simulink model "MyComplexModel_V13R2023a"  (R2023a)
settings: Solver=ode23tb  StartTime=0.0  StopTime=30  FixedStep=0.001  MaxStep=0.001  RelTol=1e-6
values from neighbouring files (symbols this model uses):
  alpha_IS = 30 / (V30_IS.^beta_IS)    [run_one_case_conditional_sampling_pediatric_noVAD_linear.m]    (also in run_one_case_pediatric_noVAD_linear.m)
  alpha_LA = 30 / (V30_LA.^beta_LA)    [run_one_case_conditional_sampling_pediatric_noVAD_linear.m]    (also in run_one_case_pediatric_noVAD_linear.m)
  alpha_LV = 30 / (V30_LV.^beta_LV)    [run_one_case_conditional_sampling_pediatric_noVAD_linear.m]    (also in run_one_case_pediatric_noVAD_linear.m)
  alpha_RA = 30 / (V30_RA.^beta_RA)    [run_one_case_conditional_sampling_pediatric_noVAD_linear.m]    (also in run_one_case_pediatric_noVAD_linear.m)
  alpha_RV = 30 / (V30_RV.^beta_RV)    [run_one_case_conditional_sampling_pediatric_noVAD_linear.m]    (also in run_one_case_pediatric_noVAD_linear.m)
  beta_IS = (log(Pm_IS / 30)) / (log(Vm_IS / V30_IS))    [run_one_case_conditional_sampling_pediatric_noVAD_linear.m]    (also in run_one_case_pediatric_noVAD_linear.m)
  beta_LA = (log(Pm_LA / 30)) / (log(Vm_LA / V30_LA))    [run_one_case_conditional_sampling_pediatric_noVAD_linear.m]    (also in run_one_case_pediatric_noVAD_linear.m)
  beta_LV = (log(Pm_LV / 30)) / (log(Vm_LV / V30_LV))    [run_one_case_conditional_sampling_pediatric_noVAD_linear.m]    (also in run_one_case_pediatric_noVAD_linear.m)
  beta_RA = (log(Pm_RA / 30)) / (log(Vm_RA / V30_RA))    [run_one_case_conditional_sampling_pediatric_noVAD_linear.m]    (also in run_one_case_pediatric_noVAD_linear.m)
  beta_RV = (log(Pm_RV / 30)) / (log(Vm_RV / V30_RV))    [run_one_case_conditional_sampling_pediatric_noVAD_linear.m]    (also in run_one_case_pediatric_noVAD_linear.m)
  C_can_H = 5e-6    (= 5e-06)    [run_one_case_conditional_sampling_pediatric_noVAD_linear.m]    (also in run_one_case_pediatric_noVAD_linear.m)
  Cla = 1.6 * 2    (= 3.2)    [run_one_case_conditional_sampling_pediatric_noVAD_linear.m]    (also in run_one_case_pediatric_noVAD_linear.m)
  Cpulmart = SV_RV / (sPAP - dPAP) * 0.65    [run_one_case_conditional_sampling_pediatric_noVAD_linear.m]    (also in run_one_case_pediatric_noVAD_linear.m = 0.830555555556)
  Cpulmven = Cpulm - Cpulmart    [run_one_case_conditional_sampling_pediatric_noVAD_linear.m]    (also in run_one_case_pediatric_noVAD_linear.m)
  Cra = 4.2 * 2    (= 8.4)    [run_one_case_conditional_sampling_pediatric_noVAD_linear.m]    (also in run_one_case_pediatric_noVAD_linear.m)
  Csysart = SV_LV / (SAP - DAP)    [run_one_case_conditional_sampling_pediatric_noVAD_linear.m]    (also in run_one_case_pediatric_noVAD_linear.m = 0.589743589744)
  Csysven = Csys - Csysart    [run_one_case_conditional_sampling_pediatric_noVAD_linear.m]    (also in run_one_case_pediatric_noVAD_linear.m)
  DE = 2 * 0    (= 0)    [run_one_case_conditional_sampling_pediatric_noVAD_linear.m]    (also in run_one_case_pediatric_noVAD_linear.m)
  DR = 3 * 0    (= 0)    [run_one_case_conditional_sampling_pediatric_noVAD_linear.m]    (also in run_one_case_pediatric_noVAD_linear.m)
  DTs = 3 * 0    (= 0)    [run_one_case_conditional_sampling_pediatric_noVAD_linear.m]    (also in run_one_case_pediatric_noVAD_linear.m)
  DTv = 0.5 * 0    (= 0)    [run_one_case_conditional_sampling_pediatric_noVAD_linear.m]    (also in run_one_case_pediatric_noVAD_linear.m)
  DV = 5 * 0    (= 0)    [run_one_case_conditional_sampling_pediatric_noVAD_linear.m]    (also in run_one_case_pediatric_noVAD_linear.m)
  Emax_LV = 0.5    [run_one_case_conditional_sampling_pediatric_noVAD_linear.m]    (also in run_one_case_pediatric_noVAD_linear.m)
  Emax_RV = 0.5    [run_one_case_conditional_sampling_pediatric_noVAD_linear.m]    (also in run_one_case_pediatric_noVAD_linear.m)
  Emin_LV = -0.5    [run_one_case_conditional_sampling_pediatric_noVAD_linear.m]    (also in run_one_case_pediatric_noVAD_linear.m)
  Emin_RV = -0.5    [run_one_case_conditional_sampling_pediatric_noVAD_linear.m]    (also in run_one_case_pediatric_noVAD_linear.m)
  ESP_LA = LAP * 1.2    [run_one_case_conditional_sampling_pediatric_noVAD_linear.m]    (also in run_one_case_pediatric_noVAD_linear.m = 22.8)
  ESP_LV = k_ESP_LV * SAP    [run_one_case_conditional_sampling_pediatric_noVAD_linear.m]    (also in run_one_case_pediatric_noVAD_linear.m)
  ESP_RA = CVP * 1.2    [run_one_case_conditional_sampling_pediatric_noVAD_linear.m]    (also in run_one_case_pediatric_noVAD_linear.m = 12)
  ESP_RV = k_ESP_RV * sPAP    [run_one_case_conditional_sampling_pediatric_noVAD_linear.m]    (also in run_one_case_pediatric_noVAD_linear.m)
  ESV_LA = EDV_LA - SV_LA    [run_one_case_conditional_sampling_pediatric_noVAD_linear.m]    (also in run_one_case_pediatric_noVAD_linear.m = 59.75)
  ESV_LV = get_required_scalar(sample_row, {'ESVLV', 'ESV_LV'})    [run_one_case_conditional_sampling_pediatric_noVAD_linear.m]    (also in run_one_case_pediatric_noVAD_linear.m = 76)
  ESV_RA = EDV_RA - SV_RA    [run_one_case_conditional_sampling_pediatric_noVAD_linear.m]    (also in run_one_case_pediatric_noVAD_linear.m = 30.05)
  ESV_RV = get_required_scalar(sample_row, {'ESVRV', 'ESV_RV'})    [run_one_case_conditional_sampling_pediatric_noVAD_linear.m]    (also in run_one_case_pediatric_noVAD_linear.m = 40)
  GaE = 0.012    [run_one_case_conditional_sampling_pediatric_noVAD_linear.m]    (also in run_one_case_pediatric_noVAD_linear.m)
  GaR = 0.1    [run_one_case_conditional_sampling_pediatric_noVAD_linear.m]    (also in run_one_case_pediatric_noVAD_linear.m)
  GaTs = 0.015    [run_one_case_conditional_sampling_pediatric_noVAD_linear.m]    (also in run_one_case_pediatric_noVAD_linear.m)
  GaTv = 0.028    [run_one_case_conditional_sampling_pediatric_noVAD_linear.m]    (also in run_one_case_pediatric_noVAD_linear.m)
  GaV = 9.29    [run_one_case_conditional_sampling_pediatric_noVAD_linear.m]    (also in run_one_case_pediatric_noVAD_linear.m)
  GpE = 0    [run_one_case_conditional_sampling_pediatric_noVAD_linear.m]    (also in run_one_case_pediatric_noVAD_linear.m)
  GpR = 0.33    [run_one_case_conditional_sampling_pediatric_noVAD_linear.m]    (also in run_one_case_pediatric_noVAD_linear.m)
  GpTs = 0    [run_one_case_conditional_sampling_pediatric_noVAD_linear.m]    (also in run_one_case_pediatric_noVAD_linear.m)
  GpTv = 0.25    [run_one_case_conditional_sampling_pediatric_noVAD_linear.m]    (also in run_one_case_pediatric_noVAD_linear.m)
  GpV = 0    [run_one_case_conditional_sampling_pediatric_noVAD_linear.m]    (also in run_one_case_pediatric_noVAD_linear.m)
  hr = get_required_scalar(sample_row, {'hr'})    [run_one_case_conditional_sampling_pediatric_noVAD_linear.m]    (also in run_one_case_pediatric_noVAD_linear.m = 112)
  kELV = (Emax_LV - Emin_LV) / (4 * SE0)    (= 0.25)    [run_one_case_conditional_sampling_pediatric_noVAD_linear.m]    (also in run_one_case_pediatric_noVAD_linear.m)
  kERV = (Emax_RV - Emin_RV) / (4 * SE0)    (= 0.25)    [run_one_case_conditional_sampling_pediatric_noVAD_linear.m]    (also in run_one_case_pediatric_noVAD_linear.m)
  kR = (Rmax - Rmin) / (4 * SR0)    (= 0.174809457508)    [run_one_case_conditional_sampling_pediatric_noVAD_linear.m]    (also in run_one_case_pediatric_noVAD_linear.m)
  kT = (Tmax - Tmin) / (4 * ST0)    (= 0.252)    [run_one_case_conditional_sampling_pediatric_noVAD_linear.m]    (also in run_one_case_pediatric_noVAD_linear.m)
  kV = (Vmax - Vmin) / (4 * SV0) / 100    (= 1.75)    [run_one_case_conditional_sampling_pediatric_noVAD_linear.m]    (also in run_one_case_pediatric_noVAD_linear.m)
  L = 1e-6    (= 1e-06)    [Simulink_vars_code.m]    (also in run_one_case_conditional_sampling_pediatric_noVAD_linear.m; run_one_case_pediatric_noVAD_linear.m)
  Lav = Lav / fct    (= 5.64234254909e-06)    [run_one_case_conditional_sampling_pediatric_noVAD_linear.m]    (also in run_one_case_pediatric_noVAD_linear.m)
  Lmv = Lmv / fct    (= 3.13989149577e-06)    [run_one_case_conditional_sampling_pediatric_noVAD_linear.m]    (also in run_one_case_pediatric_noVAD_linear.m)
  Lpv = Lpv / fct    (= 5.14307516405e-06)    [run_one_case_conditional_sampling_pediatric_noVAD_linear.m]    (also in run_one_case_pediatric_noVAD_linear.m)
  Ltv = Ltv / fct    (= 2.29209519806e-06)    [run_one_case_conditional_sampling_pediatric_noVAD_linear.m]    (also in run_one_case_pediatric_noVAD_linear.m)
  mcfp = CO / 60 * Rsysven + CVP    [run_one_case_conditional_sampling_pediatric_noVAD_linear.m]    (also in run_one_case_pediatric_noVAD_linear.m)
  Poffset_IS = Poffset_LV    (= 0)    [run_one_case_conditional_sampling_pediatric_noVAD_linear.m]    (also in run_one_case_pediatric_noVAD_linear.m)
  Poffset_LA = 0    [run_one_case_conditional_sampling_pediatric_noVAD_linear.m]    (also in run_one_case_pediatric_noVAD_linear.m)
  Poffset_LV = 0    [run_one_case_conditional_sampling_pediatric_noVAD_linear.m]    (also in run_one_case_pediatric_noVAD_linear.m)
  Poffset_RA = 0    [run_one_case_conditional_sampling_pediatric_noVAD_linear.m]    (also in run_one_case_pediatric_noVAD_linear.m)
  Poffset_RV = 0    [run_one_case_conditional_sampling_pediatric_noVAD_linear.m]    (also in run_one_case_pediatric_noVAD_linear.m)
  Ps_IS = Ps_LV    [run_one_case_conditional_sampling_pediatric_noVAD_linear.m]    (also in run_one_case_pediatric_noVAD_linear.m)
  Ps_LA = ESP_LA    [run_one_case_conditional_sampling_pediatric_noVAD_linear.m]    (also in run_one_case_pediatric_noVAD_linear.m = 22.8)
  Ps_LV = ESP_LV    [run_one_case_conditional_sampling_pediatric_noVAD_linear.m]    (also in run_one_case_pediatric_noVAD_linear.m)
  Ps_RA = ESP_RA    [run_one_case_conditional_sampling_pediatric_noVAD_linear.m]    (also in run_one_case_pediatric_noVAD_linear.m = 12)
  Ps_RV = ESP_RV    [run_one_case_conditional_sampling_pediatric_noVAD_linear.m]    (also in run_one_case_pediatric_noVAD_linear.m)
  R = 1e-6    (= 1e-06)    [Simulink_vars_code.m]    (also in run_one_case_conditional_sampling_pediatric_noVAD_linear.m; run_one_case_pediatric_noVAD_linear.m)
  Rdir_AV = 0.00375    [run_one_case_conditional_sampling_pediatric_noVAD_linear.m]    (also in run_one_case_pediatric_noVAD_linear.m)
  Rdir_MV = 0.0075    [run_one_case_conditional_sampling_pediatric_noVAD_linear.m]    (also in run_one_case_pediatric_noVAD_linear.m)
  Rdir_PV = 0.00375    [run_one_case_conditional_sampling_pediatric_noVAD_linear.m]    (also in run_one_case_pediatric_noVAD_linear.m)
  Rdir_TV = 0.00375    [run_one_case_conditional_sampling_pediatric_noVAD_linear.m]    (also in run_one_case_pediatric_noVAD_linear.m)
  Rinv_AV = 50    [run_one_case_conditional_sampling_pediatric_noVAD_linear.m]    (also in run_one_case_pediatric_noVAD_linear.m)
  Rinv_MV = 50    [run_one_case_conditional_sampling_pediatric_noVAD_linear.m]    (also in run_one_case_pediatric_noVAD_linear.m)
  Rinv_PV = 50    [run_one_case_conditional_sampling_pediatric_noVAD_linear.m]    (also in run_one_case_pediatric_noVAD_linear.m)
  Rinv_TV = 50    [run_one_case_conditional_sampling_pediatric_noVAD_linear.m]    (also in run_one_case_pediatric_noVAD_linear.m)
  Rmax = (Rsp_max * Rep_max) / (Rsp_max + Rep_max)    (= 1.3359375)    [run_one_case_conditional_sampling_pediatric_noVAD_linear.m]    (also in run_one_case_pediatric_noVAD_linear.m)
  Rmin = (Rsp_min * Rep_min) / (Rsp_min + Rep_min)    (= 0.636699669967)    [run_one_case_conditional_sampling_pediatric_noVAD_linear.m]    (also in run_one_case_pediatric_noVAD_linear.m)
  rpm = 5500    [run_one_case_conditional_sampling_pediatric_noVAD_linear.m]    (also in run_one_case_pediatric_noVAD_linear.m)
  Rpulmart = k_Rpulmart * Rtotpulm    [run_one_case_conditional_sampling_pediatric_noVAD_linear.m]    (also in run_one_case_pediatric_noVAD_linear.m)
  Rpulmven = Rtotpulm - Rpulmart    [run_one_case_conditional_sampling_pediatric_noVAD_linear.m]    (also in run_one_case_pediatric_noVAD_linear.m)
  Rsysart = Rtotsys - Rsysven    [run_one_case_conditional_sampling_pediatric_noVAD_linear.m]    (also in run_one_case_pediatric_noVAD_linear.m)
  Rsysven = k_Rsysven * CO0 / CO    [run_one_case_conditional_sampling_pediatric_noVAD_linear.m]    (also in run_one_case_pediatric_noVAD_linear.m)
  st_a = 0    [conditional_sampling_generate_patients.m]    (also in run_one_case_conditional_sampling_pediatric_noVAD_linear.m; run_one_case_pediatric_noVAD_linear.m)
  st_v = 0    [conditional_sampling_generate_patients.m]    (also in run_one_case_conditional_sampling_pediatric_noVAD_linear.m; run_one_case_pediatric_noVAD_linear.m)
  st_VAD = 0    [conditional_sampling_generate_patients.m]    (also in run_one_case_conditional_sampling_pediatric_noVAD_linear.m; run_one_case_pediatric_noVAD_linear.m)
  st_VADtype = 0    [run_one_case_conditional_sampling_pediatric_noVAD_linear.m]    (also in run_one_case_pediatric_noVAD_linear.m)
  TauE = 1.5    [run_one_case_conditional_sampling_pediatric_noVAD_linear.m]    (also in run_one_case_pediatric_noVAD_linear.m)
  TauR = 1.5    [run_one_case_conditional_sampling_pediatric_noVAD_linear.m]    (also in run_one_case_pediatric_noVAD_linear.m)
  TauTs = 1.8    [run_one_case_conditional_sampling_pediatric_noVAD_linear.m]    (also in run_one_case_pediatric_noVAD_linear.m)
  TauTv = 0.8    [run_one_case_conditional_sampling_pediatric_noVAD_linear.m]    (also in run_one_case_pediatric_noVAD_linear.m)
  TauV = 10    [run_one_case_conditional_sampling_pediatric_noVAD_linear.m]    (also in run_one_case_pediatric_noVAD_linear.m)
  Te = Tresp - Ti    (= 3)    [run_one_case_conditional_sampling_pediatric_noVAD_linear.m]    (also in run_one_case_pediatric_noVAD_linear.m)
  Ti = 2    [run_one_case_conditional_sampling_pediatric_noVAD_linear.m]    (also in run_one_case_pediatric_noVAD_linear.m)
  Tmax = 1.308    [run_one_case_conditional_sampling_pediatric_noVAD_linear.m]    (also in run_one_case_pediatric_noVAD_linear.m)
  Tmin = 0.3    [run_one_case_conditional_sampling_pediatric_noVAD_linear.m]    (also in run_one_case_pediatric_noVAD_linear.m)
  Tresp = 5    [run_one_case_conditional_sampling_pediatric_noVAD_linear.m]    (also in run_one_case_pediatric_noVAD_linear.m)
  V0_LA = 0    [run_one_case_conditional_sampling_pediatric_noVAD_linear.m]    (also in run_one_case_pediatric_noVAD_linear.m)
  V0_LV = 0    [run_one_case_conditional_sampling_pediatric_noVAD_linear.m]    (also in run_one_case_pediatric_noVAD_linear.m)
  V0_RA = 0    [run_one_case_conditional_sampling_pediatric_noVAD_linear.m]    (also in run_one_case_pediatric_noVAD_linear.m)
  V0_RV = 0    [run_one_case_conditional_sampling_pediatric_noVAD_linear.m]    (also in run_one_case_pediatric_noVAD_linear.m)
  Vd_IS = Vd_LV * 0.1    (= 0)    [run_one_case_conditional_sampling_pediatric_noVAD_linear.m]    (also in run_one_case_pediatric_noVAD_linear.m)
  Vd_LA = 0    [run_one_case_conditional_sampling_pediatric_noVAD_linear.m]    (also in run_one_case_pediatric_noVAD_linear.m)
  Vd_LV = 0    [run_one_case_conditional_sampling_pediatric_noVAD_linear.m]    (also in run_one_case_pediatric_noVAD_linear.m)
  Vd_RA = 0    [run_one_case_conditional_sampling_pediatric_noVAD_linear.m]    (also in run_one_case_pediatric_noVAD_linear.m)
  Vd_RV = 0    [run_one_case_conditional_sampling_pediatric_noVAD_linear.m]    (also in run_one_case_pediatric_noVAD_linear.m)
  Vmax = Vusv_max + Vuev_max    (= 2846)    [run_one_case_conditional_sampling_pediatric_noVAD_linear.m]    (also in run_one_case_pediatric_noVAD_linear.m)
  Vmin = Vusv_min + Vuev_min    (= 2146)    [run_one_case_conditional_sampling_pediatric_noVAD_linear.m]    (also in run_one_case_pediatric_noVAD_linear.m)
  Vs_IS = Vs_LV * 0.1    [run_one_case_conditional_sampling_pediatric_noVAD_linear.m]    (also in run_one_case_pediatric_noVAD_linear.m = 11.4)
  Vs_LA = EDV_LA + 5    [run_one_case_conditional_sampling_pediatric_noVAD_linear.m]    (also in run_one_case_pediatric_noVAD_linear.m = 69.35)
  Vs_LV = EDV_LV + 15    [run_one_case_conditional_sampling_pediatric_noVAD_linear.m]    (also in run_one_case_pediatric_noVAD_linear.m = 114)
  Vs_RA = EDV_RA + 5    [run_one_case_conditional_sampling_pediatric_noVAD_linear.m]    (also in run_one_case_pediatric_noVAD_linear.m = 39.65)
  Vs_RV = EDV_RV + 15    [run_one_case_conditional_sampling_pediatric_noVAD_linear.m]    (also in run_one_case_pediatric_noVAD_linear.m = 78)
  Vusv_pulm_ven = k_Vusv_pulm_ven * Vusv_pulm    [run_one_case_conditional_sampling_pediatric_noVAD_linear.m]    (also in run_one_case_pediatric_noVAD_linear.m)
  Vusv_sys_ven = k_Vusv_sys_ven * Vusv_sys    [run_one_case_conditional_sampling_pediatric_noVAD_linear.m]    (also in run_one_case_pediatric_noVAD_linear.m)
undefined symbols (not defined in the file or in its folder): magnitude
libraries: spsMeanLib x9, spsMeanVariableFrequencyLib x5, simulink x3, dspsigops x1
(part 1 of 2)
settings Model: Creator=luger  LastModifiedBy=Admin
settings DataIOCC: ExternalInput=getinputstruct(op1)  InitialState=getstatestruct(op1)  SaveFormat=Array  DatasetSignalFormat=timetable
settings RTWCC: GPUComputeCapability=5.0

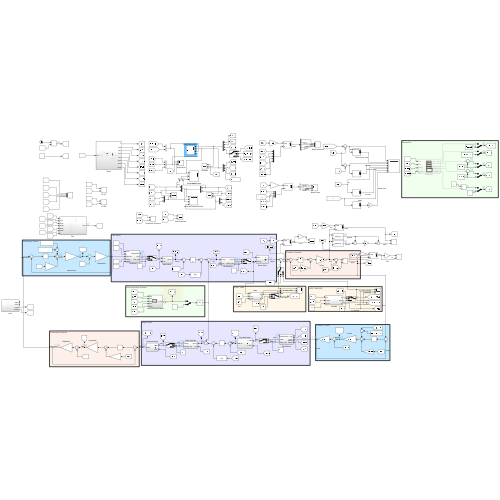
[thumbnail: Simulink's stored preview of the top-level diagram]
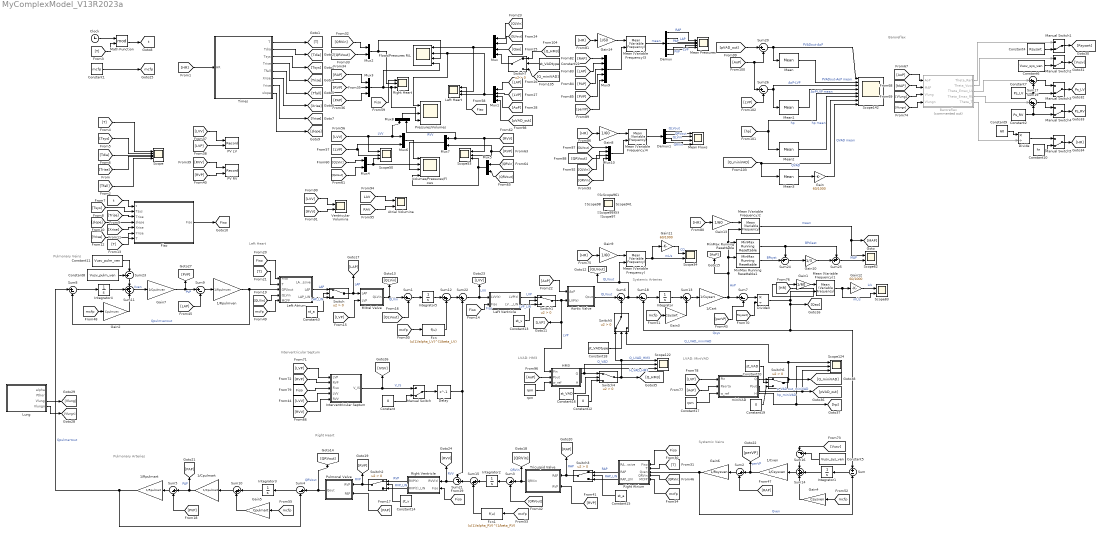
== system MyComplexModel_V13R2023a ==
  note: LVAD: MiniVAD
  note: LVAD: HM3
  note: Interventricular Septum
  note: Baroreflex
  note: Pulmonary Veins
  note: Pulmonary Arteries
  note: Systemic Veins
  note: Systemic Arteries
  note: Right Heart
  note: Left Heart
  1/Cart : Gain  Gain=1/Csysart
  1/Cpulmart : Gain  Gain=1/Cpulmart
  1/Cven : Gain  Gain=1/Csysven
  1/Rpulmart : Gain  Gain=1/Rpulmart
  1/Rpulmven : Gain  Gain=1/Rpulmven
  Aortic Valve : Subsystem
  Atrial Volumina : Scope  NumInputPorts=2
  Baroreflex : Subsystem  Commented=on
  Clock : Clock
  Constant : Constant  Value=0
  Constant1 : Constant  Value=mcfp
  Constant10 : Constant  Value=hr
  Constant11 : Constant  Value=Vusv_pulm_ven
  Constant12 : Constant  Value=0
  Constant13 : Constant  Value=st_v
  Constant14 : Constant  Value=st_v
  Constant15 : Constant  Value=st_a
  Constant16 : Constant  Value=st_VAD
  Constant17 : Constant  Value=rpm
  Constant18 : Constant  Value=st_VADtype
  Constant19 : Constant  Value=0
  Constant2 : Constant  Value=Ps_RV
  Constant20 : Constant  Value=st_VAD
  Constant21 : Constant  Value=st_VADtype
  Constant3 : Constant  Value=st_a
  Constant4 : Constant  Value=Rsysart
  Constant5 : Constant  Value=Vusv_sys_ven
  Constant6 : Constant  Value=Vusv_sys_ven
  Constant7 : Constant  Value=Ps_LV
  Constant8 : Constant  Value=Vusv_pulm_ven
  Constant9 : Constant  Value=60
  Delay : Delay  DelayLength=1  InitialCondition=0
  Demux : Demux  Outputs=5
  Demux1 : Demux
  Divide : Product  Inputs=*/
  Divide3 : Product  Inputs=*/
  Fcn : Fcn  Expr=(u(1)/alpha_LV)^(1/beta_LV)
  Fcn1 : Fcn  Expr=(u(1)/alpha_RV)^(1/beta_RV)
  Fiso : Subsystem
  Flows/Pressures R/L : Scope  NumInputPorts=4
  Gain : Gain  Gain=60/1000
  Gain{1,8..9,13..14} (5 alike) : Gain  Gain=1/60
  Gain10 : Gain  Gain=1/3
  Gain11 : Gain  Gain=60/1000
  Gain12 : Gain  Gain=60/1000
  Gain2 : Gain  Gain=Cpulmven
  Gain3 : Gain  Gain=Csysart
  Gain4 : Gain  Gain=Csysven
  Gain5 : Gain  Gain=Cpulmart
  Gain6 : Gain  Gain=1/Rsysven
  Gain7 : Gain  Gain=1/Cpulmven
  HM3 : Subsystem
  Integrator{,1..5} (6 alike) : Integrator
  Interventricular Septum : Subsystem
  Left Atrium : Subsystem
  Left Heart : Scope  NumInputPorts=3
  Left Ventricle : Subsystem
  Lung : Subsystem
  Manual Switch{,1..5} (6 alike) : ManualSwitch  CurrentSetting=0
  Math Function : Math  Operator=mod
  Mean{,1..3} (4 alike) : spsMeanLib/Mean  Freq=hr/60  Vinit=0  Ts=0
  Mean (Variable Frequency){,1..4} (5 alike) : spsMeanVariableFrequencyLib/Mean (Variable Frequency)  Finit=hr/60  Fmin=40/60  Vinit=0  Ts=0
      settings: LibrarySourceBlock=|
      | sps_lib/Sensors and Measurements/Mean
      | (Variable Frequency)
  Mean Flows : Scope  NumInputPorts=4
  Mean Pressures : Scope  NumInputPorts=5
  MinMax Running Resettable : simulink/Math Operations/MinMax Running Resettable  Function=min  vinit=80
  MinMax Running Resettable1 : simulink/Math Operations/MinMax Running Resettable  Function=max  vinit=2
  Mitral Valve : Subsystem
  Mux : Mux
  Mux1 : Mux
  Mux10 : Mux
  Mux{2,4..8} (6 alike) : Mux  Inputs=2
  Mux3 : Mux  Inputs=3
  Mux9 : Mux  Inputs=5
  PV LV : Record  FileSettingsInternal="{\"entries\":[{\"content\":{\"excelSettings\":{\"content\":{},\"type\":\"Streamout.ExcelSettings\"}},\"type\":\"Streamout.FileSettingStorage\",\"uuid\":\"\"}],\"packageUris\":[\"http:\\/\\/schema.mathworks.com\\/mf0\\/streamout_blocks\\/R2020a\"],\"version\":\"1.0\"}"  Layout=[1 1]  SignalsInternal="{\"entries\":[{\"content\":{\"signals\":[{\"content\":{\"blockPath\":[],\"dimensions\":[1],\"domain\":\"\",\"lineColor\":\"#64d413\",\"port\":1,\"sid\":[\"\"],\"signalID\":12905,\"signalName\":\"From37\"},\"type\":\"RecordBlkView.Signal\",\"uuid\":\"\"},{\"content\":{\"blockPath\":[],\"dimensions\":[1],\"domain\":\"\",\"lineColor\":\"#ff13a6\",\"port\":2,\"sid\":[\"\"],\"signalID\":12909,\"signalName\":\"From38\"},\"type\":\"RecordBlkView.Signal\",\"uuid\":\"\"}]},\"type\":\"RecordBlkView.InputSignals\",\"uuid\":\"\"}],\"packageUris\":[\"http:\\/\\/schema.mathworks.com\\/mf0\\/streamout_blocks\\/R2020a\"],\"version\":\"1.0\"}"  VisualizationBindings="{\"xyplotplugin\":{\"info\":[{\"series\":[],\"subplotID\":1}]}}"  CompatibilityTag=XY
  PV RV : Record  FileSettingsInternal="{\"entries\":[{\"content\":{\"excelSettings\":{\"content\":{},\"type\":\"Streamout.ExcelSettings\"}},\"type\":\"Streamout.FileSettingStorage\",\"uuid\":\"\"}],\"packageUris\":[\"http:\\/\\/schema.mathworks.com\\/mf0\\/streamout_blocks\\/R2020a\"],\"version\":\"1.0\"}"  Layout=[1 1]  SignalsInternal="{\"entries\":[{\"content\":{\"signals\":[{\"content\":{\"blockPath\":[],\"dimensions\":[1],\"domain\":\"\",\"lineColor\":\"#fe330a\",\"port\":1,\"sid\":[\"\"],\"signalID\":12913,\"signalName\":\"From39\"},\"type\":\"RecordBlkView.Signal\",\"uuid\":\"\"},{\"content\":{\"blockPath\":[],\"dimensions\":[1],\"domain\":\"\",\"lineColor\":\"#22b573\",\"port\":2,\"sid\":[\"\"],\"signalID\":12917,\"signalName\":\"From40\"},\"type\":\"RecordBlkView.Signal\",\"uuid\":\"\"}]},\"type\":\"RecordBlkView.InputSignals\",\"uuid\":\"\"}],\"packageUris\":[\"http:\\/\\/schema.mathworks.com\\/mf0\\/streamout_blocks\\/R2020a\"],\"version\":\"1.0\"}"  VisualizationBindings="{\"xyplotplugin\":{\"info\":[{\"series\":[],\"subplotID\":1}]}}"  CompatibilityTag=XY
  Pressures/Volumes : Scope  NumInputPorts=3
  Pulmonal Valve : Subsystem
  Right Atrium : Subsystem
  Right Heart : Scope  NumInputPorts=3
  Right Ventricle : Subsystem
  Scope : Scope  NumInputPorts=5
  Scope{50,53,122,124} (4 alike) : Scope  NumInputPorts=3
  Scope142 : Scope  NumInputPorts=8
  Scope34 : Scope  NumInputPorts=2
  Scope62 : Scope  NumInputPorts=2
  Scope83 : Scope  NumInputPorts=2
  Sum : Sum  Inputs=+-
  Sum{1..5,7..9,18,20,26} (11 alike) : Sum  Inputs=|+-
  Sum{6,10,12..13,15,17,19,22} (8 alike) : Sum  Inputs=|++
  Sum11 : Sum  Inputs=+++
  Sum14 : Sum  Inputs=+++
  Sum16 : Sum  Inputs=|-+
  Sum21 : Sum  Inputs=-+|
  Sum23 : Sum  Inputs=+-|
  Sum24 : Sum  Inputs=-+|
  Sum25 : Sum  Inputs=++|
  Switch{,1..7} (8 alike) : Switch  Criteria=u2 > Threshold  SaturateOnIntegerOverflow=off  InputSameDT=off
  Times : Subsystem
  Tricuspid Valve : Subsystem
  Ventricular Volumina : Scope  NumInputPorts=2
  Volumes/Pressures/Flows : Scope  NumInputPorts=4
  miniVAD : Subsystem
  rpm : Constant  Value=rpm
  Scope{1..33,35..49,51..52,54..61,63..82,84..121,123,125..141} (134 alike) : Scope
  tag scope: Fiso=global, Ps_LV=global, Ps_RV=global, mcfp=global, t=global
  wires:
  Times/5(Tfall) -> [Tfall]
  [T] -> Scope/1
  [HR] -> Times/1(HR)
  Times/3(Tsys) -> [Tsys]
  [Tsys] -> Scope/2
  [Tdia] -> Scope/3
  [Trise] -> Scope/4
  [Tfall] -> Scope/5
  Clock/1 -> Math Function/1
  [T] -> Math Function/2
  Times/8(slope) -> [slope]
  Math Function/1 -> [t]
  Times/1(T) -> [T]
  Times/2(Tdia) -> [Tdia]
  Times/4(Trise) -> [Trise]
  Times/6(Xrise) -> [Xrise]
  Times/7(Yrise) -> [Yrise]
  [t] -> Fiso/1(t)
  [Tsys] -> Fiso/2(Tsys)
  [Trise] -> Fiso/3(Trise)
  [slope] -> Fiso/4(slope)
  [Xrise] -> Fiso/5(Xrise)
  [Yrise] -> Fiso/6(Yrise)
  [T] -> Fiso/7(T)
  Fiso/1(Fiso) -> [Fiso]
  Left Ventricle/1(LVP(t)) -> Switch1/1  "LVP"
  [Fiso] -> Left Ventricle/2(Fiso)  "Fiso"
  Sum1/1 -> Integrator5/1
  Mitral Valve/1(QLVin) -> Sum1/1, [QLVin]  "QLVin"
  [QLVout] -> Sum1/2
  Aortic Valve/1(Qout) -> Sum6/1  "QLVout"
  Sum18/1 -> Integrator/1
  1/Cart/1 -> [AoP], Mean (Variable Frequency)2/2, MinMax Running Resettable/1, MinMax Running Resettable1/1, Sum7/1  "AoP"
  Sum7/1 -> Divide3/1
  Divide3/1 -> Mean (Variable Frequency)1/2, [Qao], Sum18/2, Sum/1  "Qsys"
  Mux/1 -> Left Heart/2, Flows/Pressures R/L/1
  [QLVin] -> Mux/1
  [QLVout] -> Mux/2
  [Qao] -> Mux/3
  [LAP] -> Mux1/1
  [LVP] -> Mux1/2
  Mux1/1 -> Pressures/Volumes/1, Flows/Pressures R/L/2, Left Heart/3
  [Fiso] -> Left Atrium/1(Fiso)
  [T] -> Left Atrium/2(T)
  [QLVin] -> Left Atrium/4(QLVin)
  [AoP] -> Aortic Valve/1(AoP)
  [AoP] -> Mux1/3
  [LVP] -> Mitral Valve/2(LVP)
  Sum2/1 -> Gain6/1
  [T] -> Right Atrium/2(T)
  [Fiso] -> Right Atrium/1(Fiso)
  Sum3/1 -> Integrator2/1
  Tricuspid Valve/1(QRVin) -> [QRVin], Sum3/1  "QRVin"
  [Fiso] -> Right Ventricle/2(Fiso)
  [PAP] -> Pulmonal Valve/2(PAP)
  Pulmonal Valve/1(Qout) -> [QRVout], Sum4/1  "QRVout"
  [QRVin] -> Mux2/1
  [QRVout] -> Mux2/2
  Sum4/1 -> Integrator3/1
  [PVP] -> Sum5/2
  Sum5/1 -> 1/Rpulmart/1
  1/Rpulmart/1 -> Sum8/1, Sum4/2  "Qpulmartout"
  Mux2/1 -> Flows/Pressures R/L/3, Right Heart/2
  [RAP] -> Mux3/1
  Mux3/1 -> Flows/Pressures R/L/4, Pressures/Volumes/3, Right Heart/3
  [RVP] -> Mux3/2
  [PAP] -> Mux3/3
  [LVV] -> PV LV/1
  [LVP] -> PV LV/2
  [RVV] -> PV RV/1
  [RVP] -> PV RV/2
  1/Cven/1 -> Sum2/1, [perVP]  "perVP"
  1/Cpulmart/1 -> Sum5/1, [PAP]  "PAP"
  [RVP] -> Tricuspid Valve/2(RVP)
  [QRVout] -> Sum3/2
  [perVP] -> Sum7/2
  Sum8/1 -> Integrator4/1
  Gain7/1 -> Sum9/1, [PVP]  "PVP"
  [LAP] -> Sum9/2
  Sum9/1 -> 1/Rpulmven/1
  1/Rpulmven/1 -> Left Atrium/3(QPUout), Sum8/2  "Qpulmvenout"
  Gain6/1 -> Sum/2, Right Atrium/3(Qven)  "Qven"
  [QRVin] -> Right Atrium/4(QRVin)
  Sum10/1 -> 1/Cpulmart/1
  Integrator5/1 -> Sum12/1
  Fcn/1 -> Sum12/2
  Integrator/1 -> Sum13/1
  Sum13/1 -> 1/Cart/1
  [RAP] -> Sum2/2
  Integrator2/1 -> Sum15/1
  Fcn1/1 -> Sum15/2
  [mcfp] -> Gain2/1
  [mcfp] -> Left Atrium/5(MCFP)
  [mcfp] -> Fcn/1
  Gain3/1 -> Sum13/2
  [mcfp] -> Gain3/1
  [mcfp] -> Gain4/1
  Sum/1 -> Integrator1/1
  [mcfp] -> Fcn1/1
  [mcfp] -> Right Atrium/5(MCFP)
  [mcfp] -> Gain5/1
  [LVV] -> Scope50/1, Mux6/1, Mux8/1  "LVV"
  [LVP] -> Mux6/2, Scope50/2
  [Fiso] -> Left Heart/1
  [Fiso] -> Right Heart/1
  Mux4/1 -> Volumes/Pressures/Flows/2, Scope50/3
  [QLVin] -> Mux4/1
  [QLVout] -> Mux4/2
  [QRVout] -> Mux5/2
  [QRVin] -> Mux5/1
  [RVV] -> Mux8/2, Mux7/1, Scope53/1  "RVV"
  [RVP] -> Scope53/2, Mux7/2
  Mux5/1 -> Volumes/Pressures/Flows/4, Scope53/3
  Mux6/1 -> Volumes/Pressures/Flows/1
  Mux7/1 -> Volumes/Pressures/Flows/3
  Sum15/1 -> Sum21/2
  Sum21/1 -> [RVV], Right Ventricle/1(RVV(t))  "RVV"
  Sum12/1 -> Sum22/1
  Sum22/1 -> [LVV], Left Ventricle/1(LVV(t))  "LVV"
  [LVP] -> Interventricular Septum/1(LVP)
  [RVP] -> Interventricular Septum/2(RVP)
  Constant1/1 -> [mcfp]
  [Fiso] -> Interventricular Septum/3(Fiso)
  Interventricular Septum/1(V_IS) -> [IVSV], Manual Switch/1  "V_IS"
  [LVV] -> Interventricular Septum/4(LVV)
  [RVV] -> Interventricular Septum/5(RVV)
  Constant/1 -> Manual Switch/2
  Manual Switch/1 -> Delay/1
  Lung/3(Vlung) -> [Vlung]
  [AoP] -> Baroreflex/1(AoP)
  [Vlung] -> Baroreflex/3(Vlung)
  [Vlungn] -> Baroreflex/4(Vlungn)
  Delay/1 -> Sum22/2, Sum21/1
  Baroreflex/1(Theta_Rart) -> Manual Switch1/1
  Constant4/1 -> Manual Switch1/2
  [Rsysart] -> Divide3/2
  Integrator1/1 -> Sum14/2
  Gain4/1 -> Sum14/3
  Baroreflex/2(Theta_Vusv) -> Manual Switch2/1
  Manual Switch2/1 -> [Vusv]
  Constant6/1 -> Manual Switch2/2
  Manual Switch3/1 -> [Ps_LV]
  Constant7/1 -> Manual Switch3/2, Sum17/2
  Manual Switch5/1 -> [HR]
  Constant9/1 -> Divide/1
  Baroreflex/5(Theta_T) -> Divide/2
  Gain5/1 -> Sum10/2
  Integrator3/1 -> Sum10/1
  Gain2/1 -> Sum11/3
  Integrator4/1 -> Sum11/2
  Sum14/1 -> 1/Cven/1
  Constant5/1 -> Sum16/2
  Baroreflex/3(Theta_Emax_LV) -> Sum17/1
  Sum17/1 -> Manual Switch3/1
  Sum19/1 -> Manual Switch4/1
  Manual Switch4/1 -> [Ps_RV]
  Constant2/1 -> Manual Switch4/2, Sum19/2
  Baroreflex/4(Theta_Emax_RV) -> Sum19/1
  MinMax Running Resettable/1 -> Sum24/1, Sum25/1  "BPdiast"
  MinMax Running Resettable1/1 -> Sum24/2  "BPsyst"
  Sum24/1 -> Gain10/1
  Gain10/1 -> Sum25/2
  Sum25/1 -> Scope62/2  "MAP"
  Sum11/1 -> Gain7/1  "Vven"
  Constant11/1 -> Sum23/2
  Manual Switch1/1 -> [Rsysart]
  Mean (Variable Frequency)2/1 -> Scope62/1, [MAP]  "mean"
  Divide/1 -> Manual Switch5/1
  Sum16/1 -> Sum14/1
  [Vusv] -> Sum16/1
  Lung/4(Vlungn) -> [Vlungn]
  Sum23/1 -> Sum11/1
  Constant8/1 -> Sum23/1
  Gain9/1 -> Mean (Variable Frequency)/1
  [HR] -> Gain9/1
  Mean (Variable Frequency)/1 -> Gain11/1, Scope34/2  "mL/s"
  Gain11/1 -> Scope34/1  "CO"
  Constant10/1 -> Manual Switch5/2
  Mean (Variable Frequency)1/1 -> Gain12/1, Scope83/2  "mL/s"
  Gain12/1 -> Scope83/1  "L/s"
  [HR] -> Gain1/1
  Gain1/1 -> Mean (Variable Frequency)1/1
  [HR] -> Gain13/1
  Gain13/1 -> Mean (Variable Frequency)2/1
  [MAP] -> Baroreflex/2(MAP)
  [HR] -> Gain14/1
  Gain14/1 -> Mean (Variable Frequency)3/1
  [RAP] -> Mux9/1
  [LAP] -> Mux9/2
  [PAP] -> Mux9/3
  [PVP] -> Mux9/4
  Mux9/1 -> Mean (Variable Frequency)3/2
  Mean (Variable Frequency)3/1 -> Demux/1  "mean"
  Demux/1 -> Mean Pressures/1  "RAP"
  Demux/2 -> Mean Pressures/2  "LAP"
  Demux/3 -> Mean Pressures/3  "PAP"
  Demux/4 -> Mean Pressures/4  "PVP"
  [HR] -> Gain8/1
  Gain8/1 -> Mean (Variable Frequency)4/1
  [QLVout] -> Mux10/1
  [QRVout] -> Mux10/2
  Mux10/1 -> Mean (Variable Frequency)4/2
  Mean (Variable Frequency)4/1 -> Demux1/1
  Demux1/1 -> Mean Flows/1  "QLVout"
  Demux1/2 -> Mean Flows/2  "QRVout"
  [perVP] -> Mux9/5
  Demux/5 -> Mean Pressures/5  "CVP"
  [LVV] -> Ventricular Volumina/1
  [RVV] -> Ventricular Volumina/2
  [QLVin] -> Mux10/3
  [QRVin] -> Mux10/4
  Demux1/3 -> Mean Flows/3  "QLVin"
  Demux1/4 -> Mean Flows/4  "QRVin"
  [LAV] -> Atrial Volumina/1
  [RAV] -> Atrial Volumina/2
  Switch1/1 -> HM3/1(Pin), [LVP], Aortic Valve/2(LVP(t))  "LVP"
  Left Ventricle/2(LVP(t)_LIN) -> Switch1/3  "LVP_LIN"
  Switch2/1 -> [RVP], Pulmonal Valve/1(RVP)  "RVP"
  Right Ventricle/2(RVP(t)_LIN) -> Switch2/3  "RVP_LIN"
  Right Ventricle/1(RVP(t)) -> Switch2/1  "RVP"
  Right Atrium/3(RAP_LIN) -> Switch3/3  "RAP_LIN"
  Right Atrium/2(RAP) -> Switch3/1  "RAP"
  Switch3/1 -> [RAP], Tricuspid Valve/1(RAP)  "RAP"
  Switch/1 -> Mitral Valve/1(LAP), [LAP]  "LAP"
  Left Atrium/2(LAP) -> Switch/1  "LAP"
  Left Atrium/3(LAP_LIN) -> Switch/3  "LAP_LIN"
  rpm/1 -> HM3/3(w_ref)
  [AoP] -> HM3/2(Pout)
  HM3/1(Q) -> Switch4/1, Scope122/2  "Q_VAD"
  Switch4/1 -> Switch5/1, Scope122/1, [Q_HM3]  "Q_LVAD_HM3"
  HM3/2(H) -> Scope122/3  "H_VAD_HM3"
  Sum6/1 -> Mean (Variable Frequency)/2, [QLVout], Sum18/1  "QLVout"
  Constant3/1 -> Switch/2
  Constant13/1 -> Switch1/2
  Constant14/1 -> Switch2/2
  Constant15/1 -> Switch3/2
  Constant16/1 -> Switch4/2
  Constant12/1 -> Switch4/3
  miniVAD/3(H) -> Scope124/2, [hp]  "hp_miniVAD"
  miniVAD/2(Pout) -> [pVAD_out], Scope124/3  "p_VAD out_miniVAD"
  [LVP] -> miniVAD/1(Pin)
  [AoP] -> miniVAD/2(Paorta)
  Constant17/1 -> miniVAD/3(w_ref)
  Switch5/1 -> Sum6/2
  Constant18/1 -> Switch5/2
  miniVAD/1(Q) -> Switch6/1
  Switch6/1 -> Scope124/1, Switch5/3, [Q_miniVAD]  "Q_LVAD_miniVAD"
  Constant19/1 -> Switch6/3
  Constant20/1 -> Switch6/2
  Switch7/1 -> Mux/4
  [pVAD_out] -> Mux1/4
  [pVAD_out] -> Sum20/1
  [AoP] -> Sum26/1, Sum20/2
  Sum20/1 -> Mean/1, Scope142/1  "PVADout-AoP"
  Mean/1 -> Scope142/2  "PVADout-AoP mean"
  [LVP] -> Sum26/2
  Sum26/1 -> Scope142/3, Mean1/1  "AoP-LVP"
  Mean1/1 -> Scope142/4  "AoP-LVP mean"
  Mean2/1 -> Scope142/6  "hp mean"
  [hp] -> Scope142/5, Mean2/1  "hp"
  [Q_miniVAD] -> Mean3/1, Scope142/7  "QVAD"
  Mean3/1 -> Gain/1
  Gain/1 -> Scope142/8  "QVAD mean"
  Constant21/1 -> Switch7/2
  [Q_HM3] -> Switch7/1
  [Q_miniVAD] -> Switch7/3
  Mux8/1 -> Pressures/Volumes/2

== system MyComplexModel_V13R2023a/Aortic Valve ==
  AoP : Inport
  LVP(t) : Inport  Port=2
  AV Inertiance : Integrator
  Add : Sum  Inputs=+--
  Gain : Gain  Gain=1/(Lav)
  Rdir : Gain  Gain=Rdir_AV
  Rinv : Gain  Gain=Rinv_AV
  Switch : Switch  Criteria=u2 > Threshold  SaturateOnIntegerOverflow=off  InputSameDT=off
  Qout : Outport
  wires:
  Add/1 -> Gain/1
  Switch/1 -> Add/3
  LVP(t)/1 -> Add/1
  Gain/1 -> AV Inertiance/1
  AV Inertiance/1 -> Qout/1, Switch/2, Rinv/1, Rdir/1  "Qout"
  AoP/1 -> Add/2
  Rdir/1 -> Switch/1
  Rinv/1 -> Switch/3

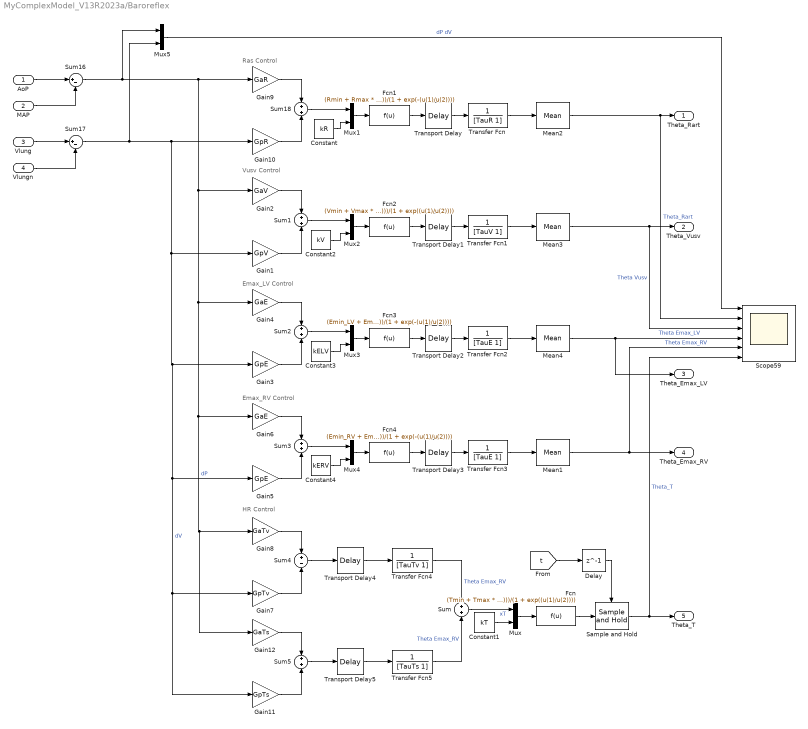
== system MyComplexModel_V13R2023a/Baroreflex ==
  note: Emax_LV Control
  note: Vusv Control
  note: Ras Control
  note: Emax_RV Control
  note: HR Control
  AoP : Inport
  MAP : Inport  Port=2
  Vlung : Inport  Port=3
  Vlungn : Inport  Port=4
  Constant : Constant  Value=kR
  Constant1 : Constant  Value=kT
  Constant2 : Constant  Value=kV
  Constant3 : Constant  Value=kELV
  Constant4 : Constant  Value=kERV
  Delay : Delay  DelayLength=1  InitialCondition=0
  Fcn : Fcn  Expr=(Tmin + Tmax * exp((u(1)/u(2))))/(1 + exp((u(1)/u(2))))
  Fcn1 : Fcn  Expr=(Rmin + Rmax * exp(-(u(1)/u(2))))/(1 + exp(-(u(1)/u(2))))
  Fcn2 : Fcn  Expr=(Vmin + Vmax * exp((u(1)/u(2))))/(1 + exp((u(1)/u(2))))
  Fcn3 : Fcn  Expr=(Emin_LV + Emax_LV * exp(-(u(1)/u(2))))/(1 + exp(-(u(1)/u(2))))
  Fcn4 : Fcn  Expr=(Emin_RV + Emax_RV * exp(-(u(1)/u(2))))/(1 + exp(-(u(1)/u(2))))
  Gain1 : Gain  Gain=GpV
  Gain10 : Gain  Gain=GpR
  Gain11 : Gain  Gain=GpTs
  Gain12 : Gain  Gain=GaTs
  Gain2 : Gain  Gain=GaV
  Gain3 : Gain  Gain=GpE
  Gain4 : Gain  Gain=GaE
  Gain5 : Gain  Gain=GpE
  Gain6 : Gain  Gain=GaE
  Gain7 : Gain  Gain=GpTv
  Gain8 : Gain  Gain=GaTv
  Gain9 : Gain  Gain=GaR
  Mean1 : spsMeanLib/Mean  Freq=hr/60  Vinit=1  Ts=0
  Mean2 : spsMeanLib/Mean  Freq=hr/60  Vinit=1  Ts=0
  Mean3 : spsMeanLib/Mean  Freq=hr/60  Vinit=Vusv_sys_ven  Ts=0
  Mean4 : spsMeanLib/Mean  Freq=hr/60  Vinit=1  Ts=0
  Mux{,1..5} (6 alike) : Mux  Inputs=2
  Sample and Hold : dspsigops/Sample and Hold  trig=Rising edge  initCond=60/hr  latchinput=off
  Scope59 : Scope  NumInputPorts=6
  Sum{,1..3,5,18} (6 alike) : Sum
  Sum16 : Sum  Inputs=|+-
  Sum17 : Sum  Inputs=|+-
  Sum4 : Sum  Inputs=+-
  Transfer Fcn : TransferFcn  Denominator=[TauR 1]
  Transfer Fcn1 : TransferFcn  Denominator=[TauV 1]
  Transfer Fcn2 : TransferFcn  Denominator=[TauE 1]
  Transfer Fcn3 : TransferFcn  Denominator=[TauE 1]
  Transfer Fcn4 : TransferFcn  Denominator=[TauTv 1]
  Transfer Fcn5 : TransferFcn  Denominator=[TauTs 1]
  Transport Delay : TransportDelay  DelayTime=DR
  Transport Delay1 : TransportDelay  DelayTime=DV
  Transport Delay2 : TransportDelay  DelayTime=DE
  Transport Delay3 : TransportDelay  DelayTime=DE
  Transport Delay4 : TransportDelay  DelayTime=DTv
  Transport Delay5 : TransportDelay  DelayTime=DTs
  Theta_Rart : Outport
  Theta_Vusv : Outport  Port=2
  Theta_Emax_LV : Outport  Port=3
  Theta_Emax_RV : Outport  Port=4
  Theta_T : Outport  Port=5
  wires:
  Gain9/1 -> Sum18/1
  Gain10/1 -> Sum18/2
  Transport Delay/1 -> Transfer Fcn/1
  Sum17/1 -> Mux5/2, Gain1/1, Gain11/1, Gain7/1, Gain5/1, Gain3/1, Gain10/1  "dV"
  Sum16/1 -> Mux5/1, Gain12/1, Gain8/1, Gain6/1, Gain4/1, Gain2/1, Gain9/1  "dP"
  Fcn1/1 -> Transport Delay/1
  AoP/1 -> Sum16/1
  MAP/1 -> Sum16/2
  Vlungn/1 -> Sum17/2
  Vlung/1 -> Sum17/1
  Transfer Fcn1/1 -> Mean3/1
  Transport Delay1/1 -> Transfer Fcn1/1
  Gain1/1 -> Sum1/2
  Gain2/1 -> Sum1/1
  Gain4/1 -> Sum2/1
  Gain3/1 -> Sum2/2
  Transfer Fcn2/1 -> Mean4/1
  Transport Delay2/1 -> Transfer Fcn2/1
  Sum2/1 -> Mux3/1
  Gain5/1 -> Sum3/2
  Transport Delay3/1 -> Transfer Fcn3/1
  Gain6/1 -> Sum3/1
  Sum3/1 -> Mux4/1
  Transfer Fcn3/1 -> Mean1/1
  Gain8/1 -> Sum4/1
  Sum4/1 -> Transport Delay4/1
  Transport Delay4/1 -> Transfer Fcn4/1
  Gain7/1 -> Sum4/2
  Sum5/1 -> Transport Delay5/1
  Transport Delay5/1 -> Transfer Fcn5/1
  Gain11/1 -> Sum5/2
  Gain12/1 -> Sum5/1
  Transfer Fcn4/1 -> Sum/1  "Theta Emax_RV"
  Transfer Fcn5/1 -> Sum/2  "Theta Emax_RV"
  Sum/1 -> Mux/1  "xT"
  Fcn/1 -> Sample and Hold/1
  Transfer Fcn/1 -> Mean2/1
  Constant1/1 -> Mux/2
  Mux/1 -> Fcn/1
  Sum18/1 -> Mux1/1
  Mux1/1 -> Fcn1/1
  Constant/1 -> Mux1/2
  Sum1/1 -> Mux2/1
  Constant2/1 -> Mux2/2
  Mux2/1 -> Fcn2/1
  Fcn2/1 -> Transport Delay1/1
  Mux3/1 -> Fcn3/1
  Fcn3/1 -> Transport Delay2/1
  Constant3/1 -> Mux3/2
  Mux4/1 -> Fcn4/1
  Fcn4/1 -> Transport Delay3/1
  Constant4/1 -> Mux4/2
  Mean2/1 -> Theta_Rart/1, Scope59/2  "Theta_Rart"
  Mean4/1 -> Theta_Emax_LV/1, Scope59/4  "Theta Emax_LV"
  Mean1/1 -> Theta_Emax_RV/1, Scope59/5  "Theta Emax_RV"
  Mean3/1 -> Theta_Vusv/1, Scope59/3  "Theta Vusv"
  [t] -> Delay/1
  Sample and Hold/1 -> Scope59/6, Theta_T/1  "Theta_T"
  Mux5/1 -> Scope59/1  "dP dV"
  Delay/1 -> Sample and Hold/Trigger

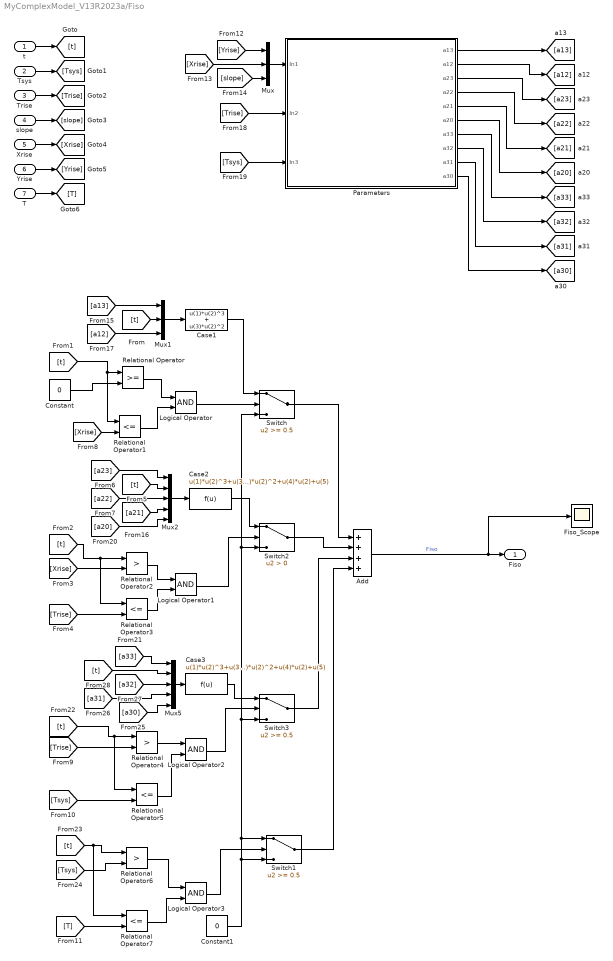
== system MyComplexModel_V13R2023a/Fiso ==
  t : Inport
  Tsys : Inport  Port=2
  Trise : Inport  Port=3
  slope : Inport  Port=4
  Xrise : Inport  Port=5
  Yrise : Inport  Port=6
  T : Inport  Port=7
  Add : Sum  Inputs=++++
  Case1 : Fcn  Expr=u(1)*u(2)^3 + u(3)*u(2)^2
  Case2 : Fcn  Expr=u(1)*u(2)^3+u(3)*u(2)^2+u(4)*u(2)+u(5)
  Case3 : Fcn  Expr=u(1)*u(2)^3+u(3)*u(2)^2+u(4)*u(2)+u(5)
  Constant : Constant  Value=0
  Constant1 : Constant  Value=0
  Fiso_Scope : Scope
  Logical Operator{,1..3} (4 alike) : Logic  AllPortsSameDT=off  OutDataTypeStr=boolean
  Mux : Mux  Inputs=3
  Mux1 : Mux  Inputs=3
  Mux2 : Mux  Inputs=5
  Mux5 : Mux  Inputs=5
  Parameters : Subsystem
  Relational Operator : RelationalOperator  OutDataTypeStr=boolean  RndMeth=Simplest  InputSameDT=off
  Relational Operator{1,3,5,7} (4 alike) : RelationalOperator  Operator=<=  OutDataTypeStr=boolean  RndMeth=Simplest  InputSameDT=off
  Relational Operator2 : RelationalOperator  Operator=>  OutDataTypeStr=boolean  RndMeth=Simplest  InputSameDT=off
  Relational Operator4 : RelationalOperator  Operator=>  OutDataTypeStr=boolean  RndMeth=Simplest  InputSameDT=off
  Relational Operator6 : RelationalOperator  Operator=>  OutDataTypeStr=boolean  RndMeth=Simplest  InputSameDT=off
  Switch : Switch  Threshold=0.5  SaturateOnIntegerOverflow=off  InputSameDT=off
  Switch1 : Switch  Threshold=0.5  SaturateOnIntegerOverflow=off  InputSameDT=off
  Switch2 : Switch  Criteria=u2 > Threshold  SaturateOnIntegerOverflow=off  InputSameDT=off
  Switch3 : Switch  Threshold=0.5  SaturateOnIntegerOverflow=off  InputSameDT=off
  Fiso : Outport
  wires:
  Relational Operator4/1 -> Logical Operator2/1
  Logical Operator1/1 -> Switch2/2
  [a30] -> Mux5/5
  [a13] -> Mux1/1
  [T] -> Relational Operator7/2
  Constant1/1 -> Switch1/1, Switch2/3, Switch/3, Switch3/3, Switch1/3
  Mux5/1 -> Case3/1
  Relational Operator1/1 -> Logical Operator/2
  Add/1 -> Fiso/1, Fiso_Scope/1  "Fiso"
  Case2/1 -> Switch2/1
  Relational Operator7/1 -> Logical Operator3/2
  Relational Operator5/1 -> Logical Operator2/2
  Relational Operator6/1 -> Logical Operator3/1
  Relational Operator2/1 -> Logical Operator1/1
  Case1/1 -> Switch/1
  Logical Operator/1 -> Switch/2
  Logical Operator2/1 -> Switch3/2
  [Xrise] -> Relational Operator1/2
  Relational Operator/1 -> Logical Operator/1
  [Tsys] -> Relational Operator5/2
  [Trise] -> Relational Operator4/2
  Relational Operator3/1 -> Logical Operator1/2
  [t] -> Mux1/2
  Case3/1 -> Switch3/1
  [a12] -> Mux1/3
  Constant/1 -> Relational Operator/2
  Switch2/1 -> Add/2
  [a31] -> Mux5/4
  [t] -> Mux5/2
  Mux1/1 -> Case1/1
  [a32] -> Mux5/3
  Logical Operator3/1 -> Switch1/2
  Switch3/1 -> Add/3
  Switch1/1 -> Add/4
  [Trise] -> Parameters/2(In2)
  Mux/1 -> Parameters/1(In1)
  Parameters/6(a20) -> [a20]
  Parameters/4(a22) -> [a22]
  Parameters/7(a33) -> [a33]
  Parameters/8(a32) -> [a32]
  Parameters/3(a23) -> [a23]
  Parameters/9(a31) -> [a31]
  Parameters/10(a30) -> [a30]
  [Xrise] -> Mux/2
  [Yrise] -> Mux/1
  Parameters/2(a12) -> [a12]
  Parameters/5(a21) -> [a21]
  Parameters/1(a13) -> [a13]
  [slope] -> Mux/3
  [Tsys] -> Parameters/3(In3)
  t/1 -> [t]
  Tsys/1 -> [Tsys]
  Trise/1 -> [Trise]
  slope/1 -> [slope]
  Xrise/1 -> [Xrise]
  Yrise/1 -> [Yrise]
  [t] -> Relational Operator/1, Relational Operator1/1
  Switch/1 -> Add/1
  [t] -> Relational Operator3/1, Relational Operator2/1
  [Xrise] -> Relational Operator2/2
  [Trise] -> Relational Operator3/2
  Mux2/1 -> Case2/1
  [t] -> Mux2/2
  [a23] -> Mux2/1
  [a22] -> Mux2/3
  [a21] -> Mux2/4
  [a20] -> Mux2/5
  [a33] -> Mux5/1
  [t] -> Relational Operator5/1, Relational Operator4/1
  [t] -> Relational Operator7/1, Relational Operator6/1
  [Tsys] -> Relational Operator6/2
  T/1 -> [T]

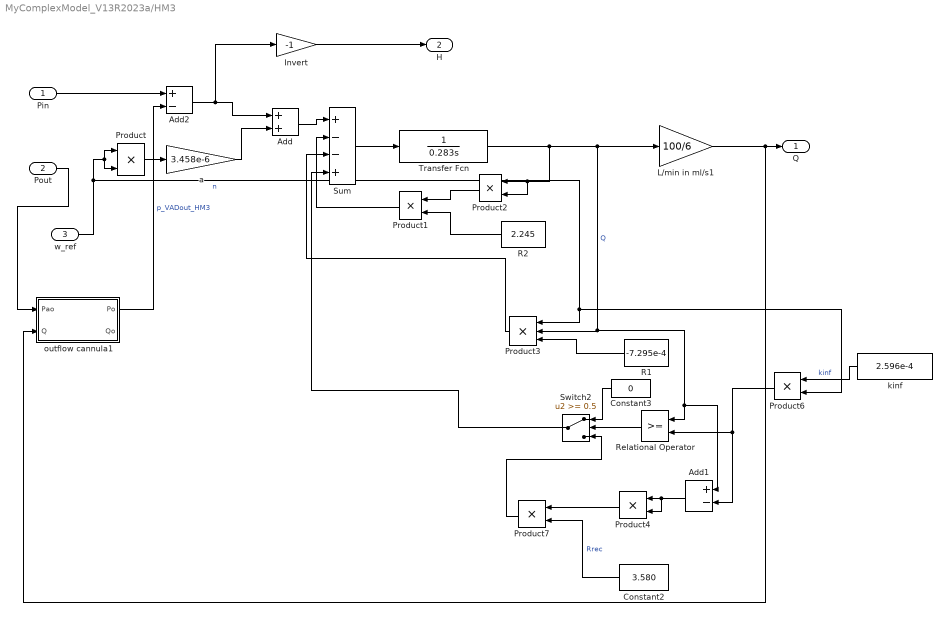
== system MyComplexModel_V13R2023a/HM3 ==
  Pin : Inport
  Pout : Inport  Port=2
  w_ref : Inport  Port=3
  Add : Sum
  Add1 : Sum  Inputs=+-
  Add2 : Sum  Inputs=+-
  Constant2 : Constant  Value=3.580
  Constant3 : Constant  Value=0
  Invert : Gain  Gain=-1
  L/min in ml/s1 : Gain  Gain=100/6
  Product{,1..2,4,6..7} (6 alike) : Product  RndMeth=Zero
  Product3 : Product  Inputs=3  RndMeth=Zero
  R1 : Constant  Value=-7.295e-4
  R2 : Constant  Value=2.245
  Relational Operator : RelationalOperator  OutDataTypeStr=boolean  RndMeth=Simplest  InputSameDT=off
  Sum : Sum  Inputs=+--+
  Switch2 : Switch  Threshold=0.5  ZeroCross=off  SaturateOnIntegerOverflow=off  InputSameDT=off
  Transfer Fcn : TransferFcn  Denominator=[0.283 0]
  a : Gain  Gain=3.458e-6
  kinf : Constant  Value=2.596e-4
  outflow cannula1 : Subsystem
  Q : Outport  VectorParamsAs1DForOutWhenUnconnected=off
  H : Outport  Port=2  VectorParamsAs1DForOutWhenUnconnected=off
  wires:
  Invert/1 -> H/1
  L/min in ml/s1/1 -> outflow cannula1/2(Q), Q/1
  Add2/1 -> Add/1, Invert/1
  outflow cannula1/1(Po) -> Add2/2  "p_VADout_HM3"
  Pout/1 -> outflow cannula1/1(Pao)
  Transfer Fcn/1 -> Product2/1, Product2/2, Product3/2, Relational Operator/1, Add1/1, L/min in ml/s1/1  "Q"
  Switch2/1 -> Sum/4
  Product7/1 -> Switch2/3
  Product4/1 -> Product7/1
  Add1/1 -> Product4/1, Product4/2
  Product6/1 -> Relational Operator/2, Add1/2
  Constant3/1 -> Switch2/1
  Relational Operator/1 -> Switch2/2
  kinf/1 -> Product6/1  "kinf"
  R2/1 -> Product1/2
  R1/1 -> Product3/3
  Constant2/1 -> Product7/2  "Rrec"
  Product3/1 -> Sum/3
  Product1/1 -> Sum/2
  Product2/1 -> Product1/1
  Sum/1 -> Transfer Fcn/1
  a/1 -> Add/2
  Pin/1 -> Add2/1
  Add/1 -> Sum/1
  w_ref/1 -> Product3/1, Product6/2, Product/2, Product/1  "n"
  Product/1 -> a/1

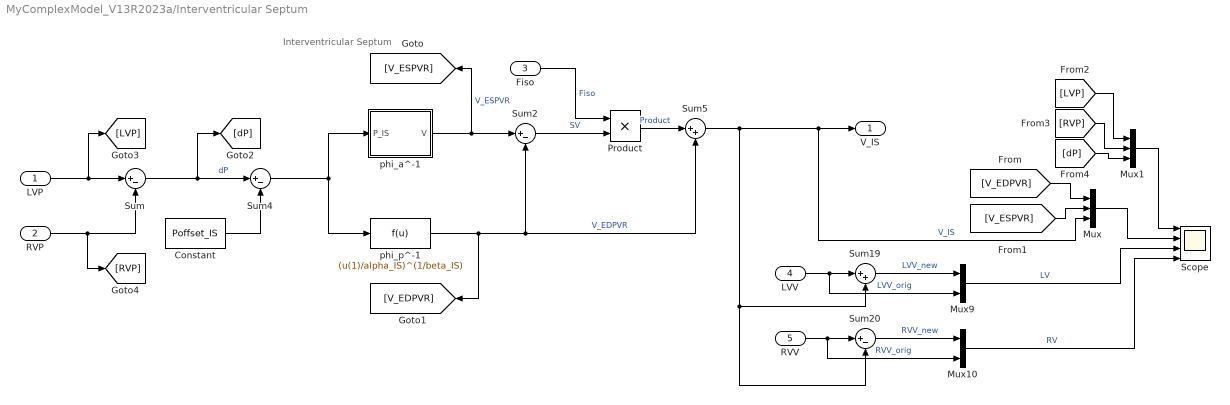
== system MyComplexModel_V13R2023a/Interventricular Septum ==
  note: Interventricular Septum
  LVP : Inport
  RVP : Inport  Port=2
  Fiso : Inport  Port=3
  LVV : Inport  Port=4
  RVV : Inport  Port=5
  Constant : Constant  Value=Poffset_IS
  Mux : Mux  Inputs=3
  Mux1 : Mux  Inputs=3
  Mux10 : Mux  Inputs=2
  Mux9 : Mux  Inputs=2
  Product : Product
  Scope : Scope  NumInputPorts=4
  Sum{,2,4,20} (4 alike) : Sum  Inputs=|+-
  Sum19 : Sum  Inputs=|++
  Sum5 : Sum  Inputs=|++
  phi_a^-1 : Subsystem
  phi_p^-1 : Fcn  Expr=(u(1)/alpha_IS)^(1/beta_IS)
  V_IS : Outport
  wires:
  Constant/1 -> Sum4/2
  Sum4/1 -> phi_p^-1/1, phi_a^-1/1(P_IS)
  phi_a^-1/1(V) -> [V_ESPVR], Sum2/1  "V_ESPVR"
  Fiso/1 -> Product/1  "Fiso"
  phi_p^-1/1 -> [V_EDPVR], Sum5/2, Sum2/2  "V_EDPVR"
  Sum2/1 -> Product/2  "SV"
  Product/1 -> Sum5/1  "Product"
  Sum5/1 -> Mux/3, V_IS/1, Sum20/2, Sum19/2  "V_IS"
  LVP/1 -> [LVP], Sum/1
  Sum/1 -> [dP], Sum4/1  "dP"
  RVP/1 -> [RVP], Sum/2
  Sum20/1 -> Mux10/1  "RVV_new"
  Mux9/1 -> Scope/3  "LV"
  Sum19/1 -> Mux9/1  "LVV_new"
  RVV/1 -> Mux10/2, Sum20/1  "RVV_orig"
  Mux10/1 -> Scope/4  "RV"
  LVV/1 -> Mux9/2, Sum19/1  "LVV_orig"
  Mux/1 -> Scope/2
  [V_EDPVR] -> Mux/1
  [V_ESPVR] -> Mux/2
  [LVP] -> Mux1/1
  Mux1/1 -> Scope/1
  [RVP] -> Mux1/2
  [dP] -> Mux1/3

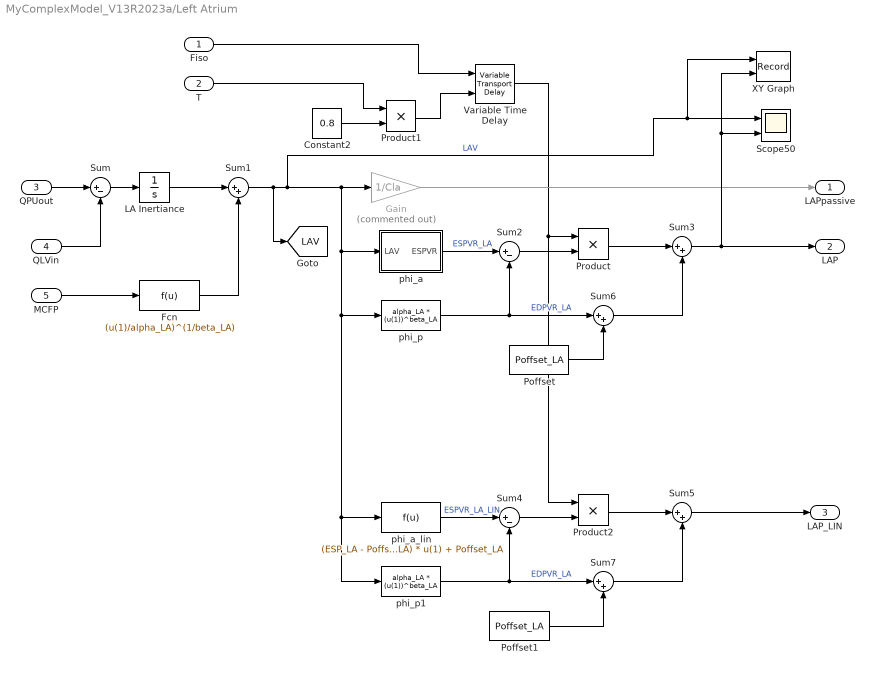
== system MyComplexModel_V13R2023a/Left Atrium ==
  Fiso : Inport
  T : Inport  Port=2
  QPUout : Inport  Port=3
  QLVin : Inport  Port=4
  MCFP : Inport  Port=5
  Constant2 : Constant  Value=0.8
  Fcn : Fcn  Expr=(u(1)/alpha_LA)^(1/beta_LA)
  Gain : Gain  Commented=on  Gain=1/Cla
  LA Inertiance : Integrator
  Poffset : Constant  Value=Poffset_LA
  Poffset1 : Constant  Value=Poffset_LA
  Product : Product
  Product1 : Product
  Product2 : Product
  Scope50 : Scope  NumInputPorts=2
  Sum : Sum  Inputs=|+-
  Sum{1,3,5..7} (5 alike) : Sum  Inputs=|++
  Sum2 : Sum  Inputs=|+-
  Sum4 : Sum  Inputs=|+-
  Variable Time Delay : VariableTransportDelay  MaximumDelay=10
  XY Graph : Record  FileSettingsInternal="{\"entries\":[{\"content\":{\"excelSettings\":{\"content\":{},\"type\":\"Streamout.ExcelSettings\"}},\"type\":\"Streamout.FileSettingStorage\",\"uuid\":\"\"}],\"packageUris\":[\"http:\\/\\/schema.mathworks.com\\/mf0\\/streamout_blocks\\/R2020a\"],\"version\":\"1.0\"}"  Layout=[1 1]  SignalsInternal="{\"entries\":[{\"content\":{\"signals\":[{\"content\":{\"blockPath\":[],\"dimensions\":[1],\"domain\":\"\",\"lineColor\":\"#139fff\",\"port\":1,\"sid\":[\"\"],\"signalID\":13061,\"signalName\":\"LAV\"},\"type\":\"RecordBlkView.Signal\",\"uuid\":\"\"},{\"content\":{\"blockPath\":[],\"dimensions\":[1],\"domain\":\"\",\"lineColor\":\"#ff6929\",\"port\":2,\"sid\":[\"\"],\"signalID\":13065,\"signalName\":\"Sum3\"},\"type\":\"RecordBlkView.Signal\",\"uuid\":\"\"}]},\"type\":\"RecordBlkView.InputSignals\",\"uuid\":\"\"}],\"packageUris\":[\"http:\\/\\/schema.mathworks.com\\/mf0\\/streamout_blocks\\/R2020a\"],\"version\":\"1.0\"}"  VisualizationBindings="{\"xyplotplugin\":{\"info\":[{\"series\":[],\"subplotID\":1}]}}"  CompatibilityTag=XY
  phi_a : Subsystem
  phi_a_lin : Fcn  Expr=(ESP_LA - Poffset_LA)/(ESV_LA - V0_LA) * u(1) + Poffset_LA
  phi_p : Fcn  Expr=alpha_LA * (u(1))^beta_LA
  phi_p1 : Fcn  Expr=alpha_LA * (u(1))^beta_LA
  LAPpassive : Outport
  LAP : Outport  Port=2
  LAP_LIN : Outport  Port=3
  tag scope: LAV=global
  wires:
  Constant2/1 -> Product1/2
  Product/1 -> Sum3/1
  phi_a/1(ESPVR) -> Sum2/1  "ESPVR_LA"
  Sum/1 -> LA Inertiance/1
  phi_p/1 -> Sum6/1, Sum2/2  "EDPVR_LA"
  Product1/1 -> Variable Time Delay/2
  Sum2/1 -> Product/2
  T/1 -> Product1/1
  Variable Time Delay/1 -> Product2/1, Product/1
  QLVin/1 -> Sum/2
  QPUout/1 -> Sum/1
  Fiso/1 -> Variable Time Delay/1
  Gain/1 -> LAPpassive/1
  LA Inertiance/1 -> Sum1/1
  MCFP/1 -> Fcn/1
  Fcn/1 -> Sum1/2
  Sum6/1 -> Sum3/2
  Poffset/1 -> Sum6/2
  Sum3/1 -> LAP/1, XY Graph/2, Scope50/2
  Sum7/1 -> Sum5/2
  Sum5/1 -> LAP_LIN/1
  Poffset1/1 -> Sum7/2
  phi_a_lin/1 -> Sum4/1  "ESPVR_LA_LIN"
  Sum1/1 -> [LAV], Gain/1, phi_a_lin/1, phi_p1/1, phi_p/1, phi_a/1(LAV), XY Graph/1, Scope50/1  "LAV"
  phi_p1/1 -> Sum7/1, Sum4/2  "EDPVR_LA"
  Product2/1 -> Sum5/1
  Sum4/1 -> Product2/2

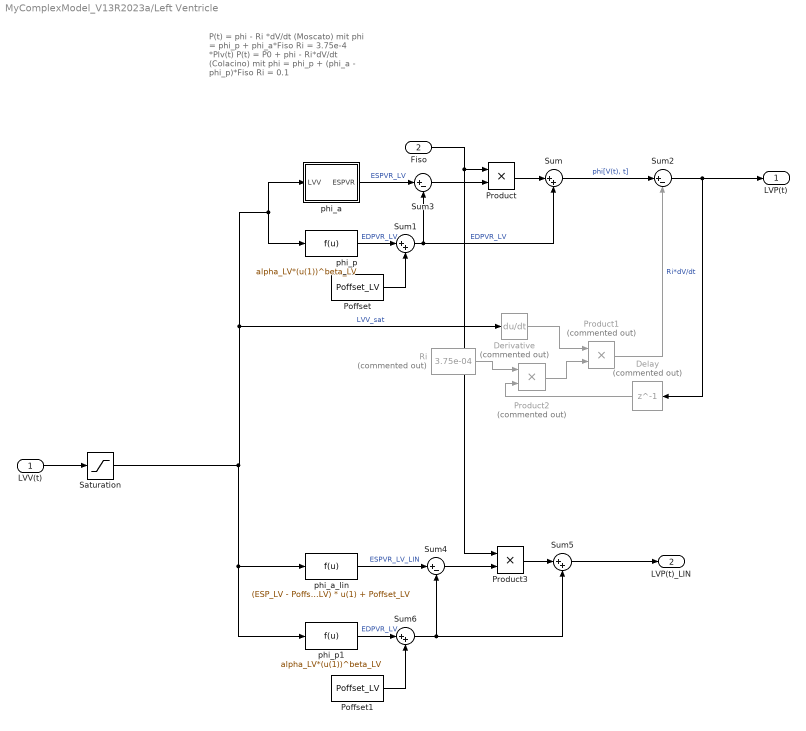
== system MyComplexModel_V13R2023a/Left Ventricle ==
  note: P(t) = phi - Ri *dV/dt (Moscato)
      | mit
      | phi = phi_p + phi_a*Fiso
      | Ri = 3.75e-4 *Plv(t)
      |
      | P(t) = P0 + phi - Ri*dV/dt (Colacino)
      | mit
      | phi = phi_p + (phi_a - phi_p)*Fiso
      | Ri = 0.1
  LVV(t) : Inport
  Fiso : Inport  Port=2
  Delay : Delay  Commented=on  DelayLength=1  InitialCondition=0
  Derivative : Derivative  Commented=on
  Poffset : Constant  Value=Poffset_LV
  Poffset1 : Constant  Value=Poffset_LV
  Product : Product
  Product1 : Product  Commented=on
  Product2 : Product  Commented=on
  Product3 : Product
  Ri : Constant  Commented=on  Value=3.75e-04
  Saturation : Saturate  UpperLimit=Inf  LowerLimit=0
  Sum{,1,5..6} (4 alike) : Sum  Inputs=|++
  Sum2 : Sum  Inputs=|+-
  Sum3 : Sum  Inputs=|+-
  Sum4 : Sum  Inputs=|+-
  phi_a : Subsystem
  phi_a_lin : Fcn  Expr=(ESP_LV - Poffset_LV)/(ESV_LV - V0_LV) * u(1) + Poffset_LV
  phi_p : Fcn  Expr=alpha_LV*(u(1))^beta_LV
  phi_p1 : Fcn  Expr=alpha_LV*(u(1))^beta_LV
  LVP(t) : Outport
  LVP(t)_LIN : Outport  Port=2
  wires:
  Poffset/1 -> Sum1/2
  Product/1 -> Sum/1
  phi_a/1(ESPVR) -> Sum3/1  "ESPVR_LV"
  LVV(t)/1 -> Saturation/1
  phi_p/1 -> Sum1/1  "EDPVR_LV"
  Fiso/1 -> Product3/1, Product/1
  Sum3/1 -> Product/2
  Sum1/1 -> Sum/2, Sum3/2  "EDPVR_LV"
  Sum/1 -> Sum2/1  "phi[V(t), t]"
  Sum2/1 -> LVP(t)/1, Delay/1
  Product1/1 -> Sum2/2  "Ri*dV/dt"
  Derivative/1 -> Product1/1
  Ri/1 -> Product2/1
  Product2/1 -> Product1/2
  Delay/1 -> Product2/2
  Saturation/1 -> phi_a_lin/1, phi_p1/1, phi_a/1(LVV), phi_p/1, Derivative/1  "LVV_sat"
  phi_a_lin/1 -> Sum4/1  "ESPVR_LV_LIN"
  phi_p1/1 -> Sum6/1  "EDPVR_LV"
  Sum4/1 -> Product3/2
  Product3/1 -> Sum5/1
  Sum6/1 -> Sum4/2, Sum5/2
  Poffset1/1 -> Sum6/2
  Sum5/1 -> LVP(t)_LIN/1
